simulink model "lump_cell_currentprofilev1_comparison"  (R2024b)
settings: Solver=FixedStepAuto  StartTime=0.0  StopTime=1320  FixedStep=0.001  RelTol=1e-3
model workspace (MAT data in the model file):
  A_busbar = 0.0015
  A_pack = 0.0059475
  C_nominal = 3
  I_max = 157.708978328
  P = 5
  S = 138
  SoC_initial = 0.769
  T_amb = 296.65
  W_max = 34
  busbar_CC_area = 0.000108
  busbar_Cp = 237
  busbar_length = 0.032
  busbar_mass = 0.01
  busbar_resistivity = 1.68e-08
  busbar_thermalcontact_resistance = 1
  cell_Cp = 1000
  cell_mass = 0.046
  h_busbar = 5
  h_pack = 5
settings Model: Creator=kara.28  LastModifiedBy=kara.28

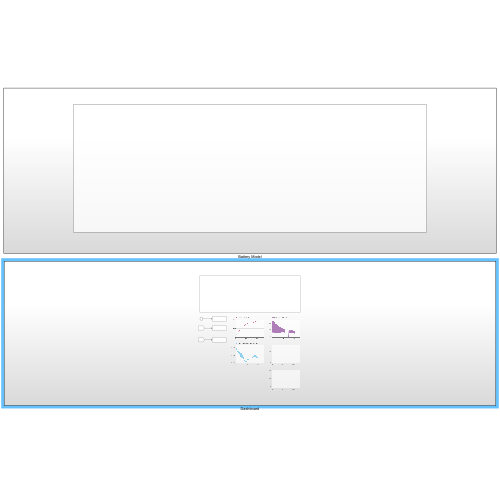
[thumbnail: Simulink's stored preview of the top-level diagram]
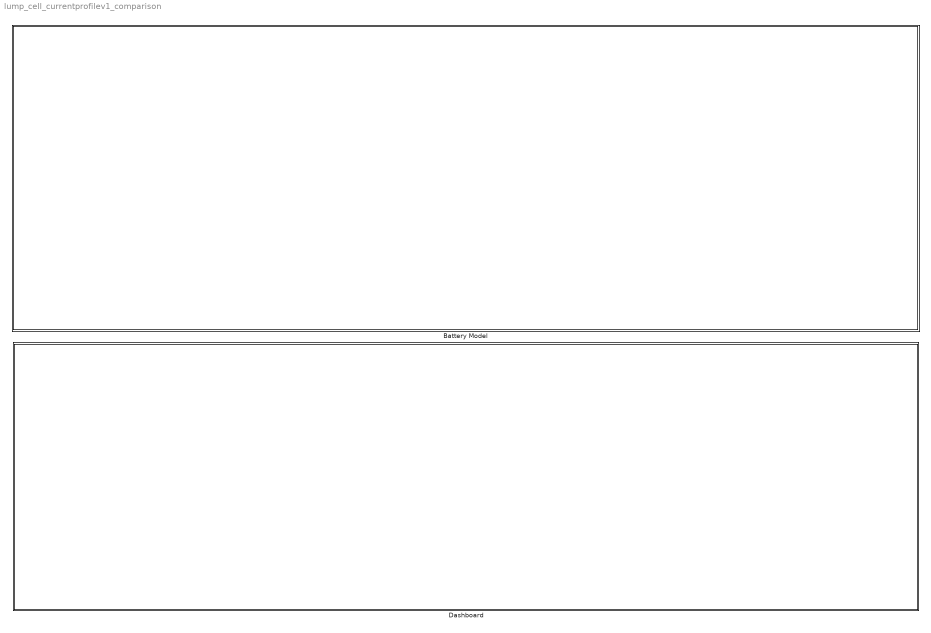
== system lump_cell_currentprofilev1_comparison ==
  Battery Model : Subsystem
  Dashboard : Subsystem

== system lump_cell_currentprofilev1_comparison/Battery Model ==
  Battery Cells : Subsystem

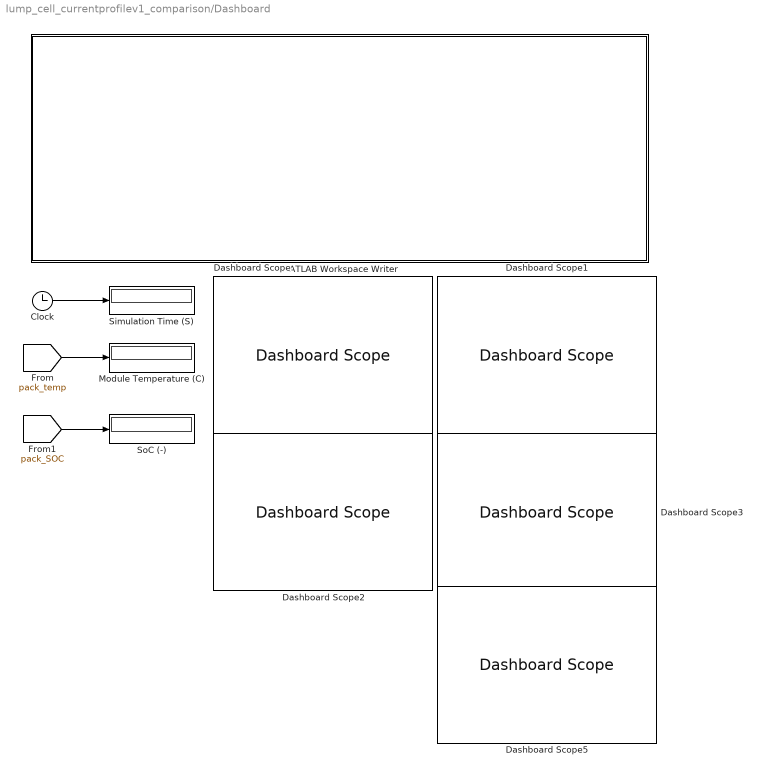
== system lump_cell_currentprofilev1_comparison/Dashboard ==
  Clock : Clock
  Dashboard Scope : DashboardScope  Ymin=35  Ymax=60
  Dashboard Scope1 : DashboardScope  Ymin=0  Ymax=180
  Dashboard Scope2 : DashboardScope
  Dashboard Scope3 : DashboardScope  Ymin=0  Ymax=1
  Dashboard Scope5 : DashboardScope
  MATLAB Workspace Writer : Subsystem
  Module Temperature (C) : Display
  Simulation Time (S) : Display
  SoC (-) : Display
  wires:
  Clock/1 -> Simulation Time (S)/1
  [pack_temp] -> Module Temperature (C)/1
  [pack_SOC] -> SoC (-)/1

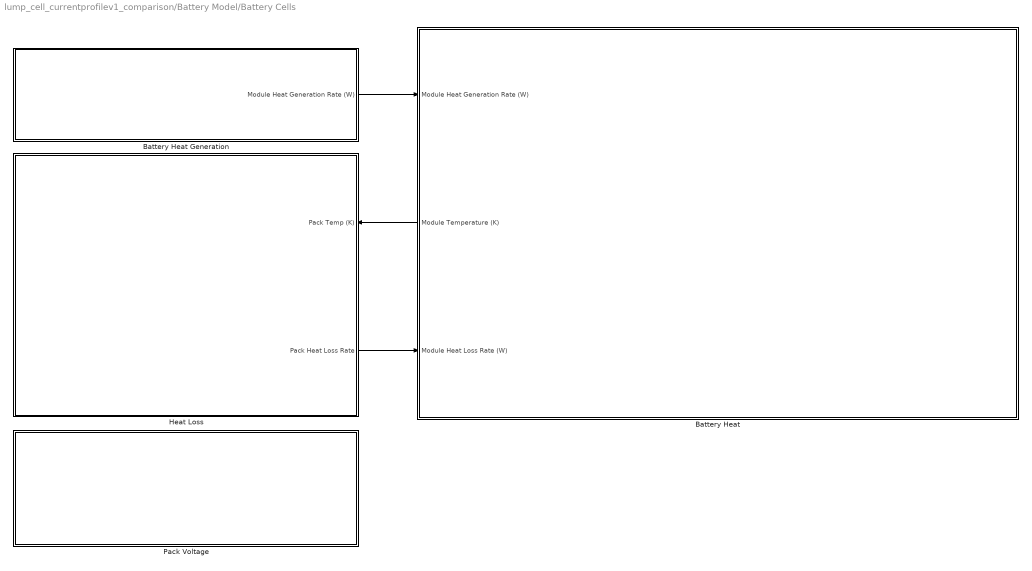
== system lump_cell_currentprofilev1_comparison/Battery Model/Battery Cells ==
  Battery Heat : Subsystem
      settings: PortSchema="{\"entries\":[{\"content\":{\"sides\":[{\"content\":{\"connectorIds\":[\"In1\",\"Out1\",\"In2\"]},\"type\":\"ConnectorPlacement.EquallySpacedRectSide\",\"uuid\":\"0f7c0562-63f7-413a-9c65-7d5d0f23ac53\"},{\"content\":{\"side\":\"RIGHT\"},\"type\":\"ConnectorPlacement.EquallySpacedRectSide\",\"uuid\":\"6856fc4a-e601-47fb-aafe-3183d6398fa2\"},{\"content\":{\"side\":\"TOP\"},\"type\":\"ConnectorPlacement.EquallySpacedRectSide\",\"uuid\":\"93500152-ab0c-4e86-a765-8796b82b9cd6\"}]},\"type\":\"ConnectorPlacement.EquallySpacedConnector\",\"uuid\":\"8bef09a8-0835-4033-ba4e-3f5f6277d0ac\"}],\"packageUris\":[\"http://schema.mathworks.com/mf0/Connector/R2020b\"],\"version\":\"1.0\"}"
  Battery Heat Generation : Subsystem
  Heat Loss : Subsystem
      settings: PortSchema="{\"entries\":[{\"content\":{\"sides\":[{\"content\":{},\"type\":\"ConnectorPlacement.EquallySpacedRectSide\",\"uuid\":\"cd11f8f0-ebc0-4dda-8c98-00f5919de41a\"},{\"content\":{\"connectorIds\":[\"In1\",\"Out1\"],\"side\":\"RIGHT\"},\"type\":\"ConnectorPlacement.EquallySpacedRectSide\",\"uuid\":\"2a68a9a1-bd97-4a17-8a8b-1aa98e9bd9a8\"},{\"content\":{\"side\":\"TOP\"},\"type\":\"ConnectorPlacement.EquallySpacedRectSide\",\"uuid\":\"debcc510-941b-4448-a371-f67c84c59f32\"}]},\"type\":\"ConnectorPlacement.EquallySpacedConnector\",\"uuid\":\"91559e46-754b-48b4-ac3e-ab135f9add0a\"}],\"packageUris\":[\"http://schema.mathworks.com/mf0/Connector/R2020b\"],\"version\":\"1.0\"}"
  Pack Voltage : Subsystem
  wires:
  Battery Heat/1(Module Temperature (K)) -> Heat Loss/1(Pack Temp (K))
  Battery Heat Generation/1(Module Heat Generation Rate (W)) -> Battery Heat/1(Module Heat Generation Rate (W))
  Heat Loss/1(Pack Heat Loss Rate) -> Battery Heat/2(Module Heat Loss Rate (W))

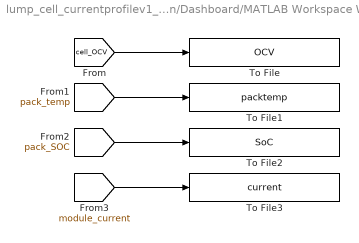
== system lump_cell_currentprofilev1_comparison/Dashboard/MATLAB Workspace Writer ==
  To File : ToFile  Filename=OCV  SampleTime=0.003
      settings: Decimation=3
  To File1 : ToFile  Filename=packtemp  SampleTime=0.003
      settings: Decimation=3
  To File2 : ToFile  Filename=SoC  SampleTime=0.003
      settings: Decimation=3
  To File3 : ToFile  Filename=current  SampleTime=0.003
      settings: Decimation=3
  wires:
  [module_current] -> To File3/1
  [cell_OCV] -> To File/1
  [pack_temp] -> To File1/1
  [pack_SOC] -> To File2/1

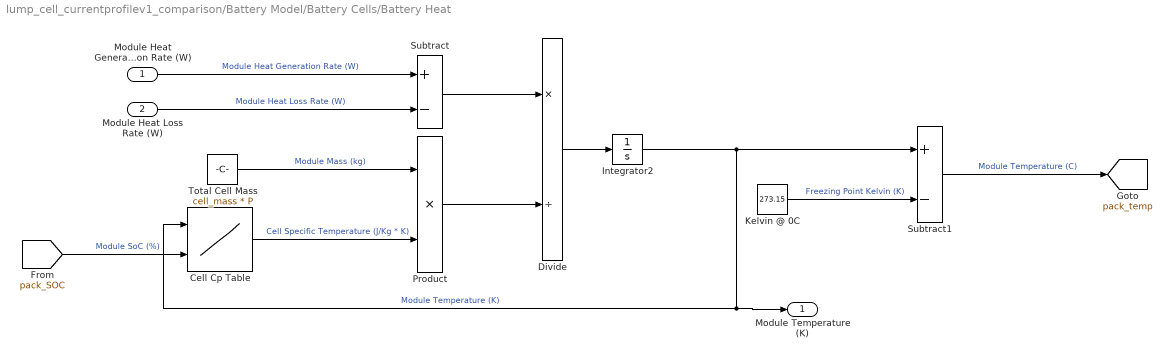
== system lump_cell_currentprofilev1_comparison/Battery Model/Battery Cells/Battery Heat ==
  Module Heat Generation Rate (W) : Inport
  Module Heat Loss Rate (W) : Inport  Port=2
  Cell Cp Table : Lookup_n-D  BreakpointsForDimension1=[296.0488;303.3425;312.147;321.5769;330.6423]  BreakpointsForDimension2=[0 0.5 1]  Table=[811.0868 819.6535 830.8545;814.1373 822.704 834.6964;817.9826 826.8129 838.6737000000001;822.2249 831.0552 843.4446;826.7299 835.8239 848.3459]  InterpMethod=Cubic spline  InternalRulePriority=Speed  RndMeth=Simplest
      settings: InputPortMap=u0,u1
  Divide : Product  Inputs=*/
  Integrator2 : Integrator  InitialCondition=T_amb
  Kelvin @ 0C : Constant  Value=273.15
  Product : Product
  Subtract : Sum  Inputs=+-
  Subtract1 : Sum  Inputs=+-
  Total Cell Mass : Constant  Value=cell_mass * P
  Module Temperature (K) : Outport
  tag scope: pack_temp=global
  wires:
  Cell Cp Table/1 -> Product/2  "Cell Specific Temperature (J/Kg * K)"
  Kelvin @ 0C/1 -> Subtract1/2  "Freezing Point Kelvin (K)"
  Divide/1 -> Integrator2/1
  Subtract/1 -> Divide/1
  Integrator2/1 -> Module Temperature (K)/1, Cell Cp Table/1, Subtract1/1  "Module Temperature (K)"
  Subtract1/1 -> [pack_temp]  "Module Temperature (C)"
  Total Cell Mass/1 -> Product/1  "Module Mass (kg)"
  Product/1 -> Divide/2
  Module Heat Loss Rate (W)/1 -> Subtract/2  "Module Heat Loss Rate (W)"
  Module Heat Generation Rate (W)/1 -> Subtract/1  "Module Heat Generation Rate (W)"
  [pack_SOC] -> Cell Cp Table/2  "Module SoC (%)"

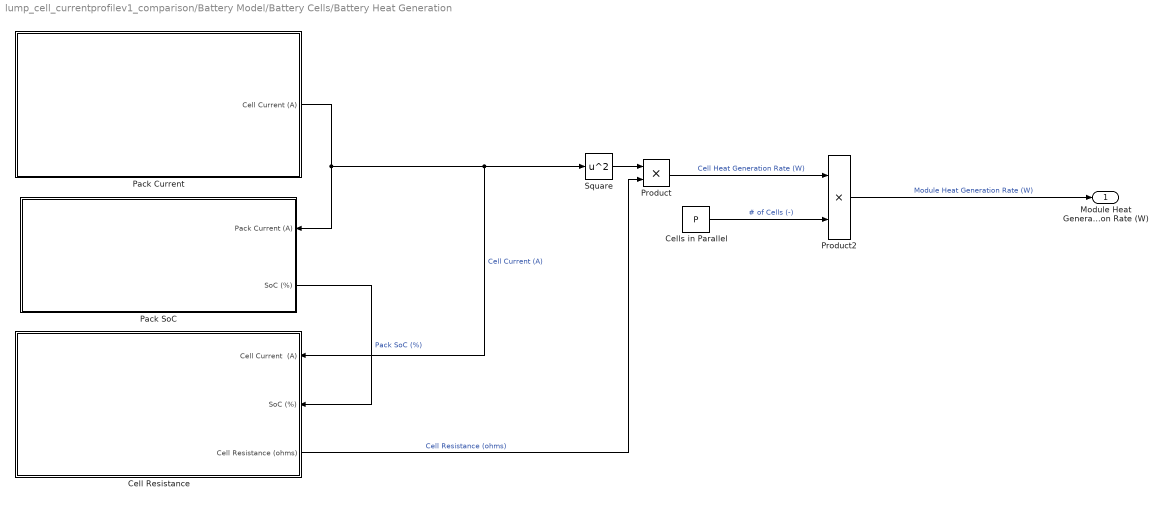
== system lump_cell_currentprofilev1_comparison/Battery Model/Battery Cells/Battery Heat Generation ==
  Cell Resistance : Subsystem
      settings: PortSchema="{\"entries\":[{\"content\":{\"sides\":[{\"content\":{},\"type\":\"ConnectorPlacement.EquallySpacedRectSide\",\"uuid\":\"1c6ff2a8-2c86-4b92-aa7d-5717a02d6f28\"},{\"content\":{\"connectorIds\":[\"In1\",\"In2\",\"Out1\"],\"side\":\"RIGHT\"},\"type\":\"ConnectorPlacement.EquallySpacedRectSide\",\"uuid\":\"52a4cb2c-e1db-459d-bd0a-206cc3bba6d1\"},{\"content\":{\"side\":\"TOP\"},\"type\":\"ConnectorPlacement.EquallySpacedRectSide\",\"uuid\":\"751bbbd6-abc7-4265-8d68-4aa70d69379f\"}]},\"type\":\"ConnectorPlacement.EquallySpacedConnector\",\"uuid\":\"b8f9630f-0167-4478-8d98-637e13782dcd\"}],\"packageUris\":[\"http://schema.mathworks.com/mf0/Connector/R2020b\"],\"version\":\"1.0\"}"
      mask Display: image('resistor.png');
  Cells in Parallel : Constant  Value=P
  Pack Current : Subsystem
      mask Display: image('current.png');
  Pack SoC : Subsystem
      settings: PortSchema="{\"entries\":[{\"content\":{\"sides\":[{\"content\":{},\"type\":\"ConnectorPlacement.EquallySpacedRectSide\",\"uuid\":\"1c6ff2a8-2c86-4b92-aa7d-5717a02d6f28\"},{\"content\":{\"connectorIds\":[\"In1\",\"Out1\"],\"side\":\"RIGHT\"},\"type\":\"ConnectorPlacement.EquallySpacedRectSide\",\"uuid\":\"52a4cb2c-e1db-459d-bd0a-206cc3bba6d1\"},{\"content\":{\"side\":\"TOP\"},\"type\":\"ConnectorPlacement.EquallySpacedRectSide\",\"uuid\":\"751bbbd6-abc7-4265-8d68-4aa70d69379f\"}]},\"type\":\"ConnectorPlacement.EquallySpacedConnector\",\"uuid\":\"b8f9630f-0167-4478-8d98-637e13782dcd\"}],\"packageUris\":[\"http://schema.mathworks.com/mf0/Connector/R2020b\"],\"version\":\"1.0\"}"
      mask Display: image('SoC.jpg');
  Product : Product
  Product2 : Product
  Square : Math  Operator=square
  Module Heat Generation Rate (W) : Outport
  wires:
  Pack Current/1(Cell Current (A)) -> Pack SoC/1(Pack Current (A)), Cell Resistance/1(Cell Current  (A)), Square/1  "Cell Current (A)"
  Cell Resistance/1(Cell Resistance (ohms)) -> Product/2  "Cell Resistance (ohms)"
  Square/1 -> Product/1
  Product/1 -> Product2/1  "Cell Heat Generation Rate (W)"
  Product2/1 -> Module Heat Generation Rate (W)/1  "Module Heat Generation Rate (W)"
  Pack SoC/1(SoC (%)) -> Cell Resistance/2(SoC (%))  "Pack SoC (%)"
  Cells in Parallel/1 -> Product2/2  "# of Cells (-)"

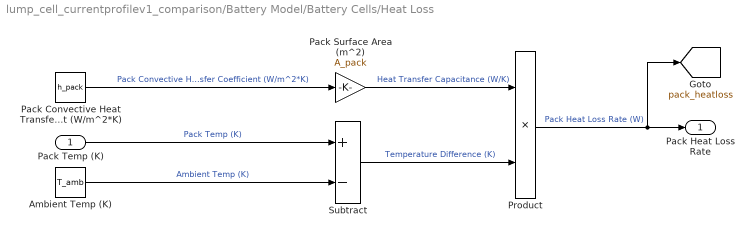
== system lump_cell_currentprofilev1_comparison/Battery Model/Battery Cells/Heat Loss ==
  Pack Temp (K) : Inport
  Ambient Temp (K) : Constant  Value=T_amb
  Pack Convective Heat Transfer Coefficient (W/m^2*K) : Constant  Value=h_pack
  Pack Surface Area (m^2) : Gain  Gain=A_pack
  Product : Product
  Subtract : Sum  Inputs=+-
  Pack Heat Loss Rate : Outport
  tag scope: pack_heatloss=global
  wires:
  Pack Convective Heat Transfer Coefficient (W/m^2*K)/1 -> Pack Surface Area (m^2)/1  "Pack Convective Heat Transfer Coefficient (W/m^2*K)"
  Subtract/1 -> Product/2  "Temperature Difference (K)"
  Pack Surface Area (m^2)/1 -> Product/1  "Heat Transfer Capacitance (W/K)"
  Product/1 -> [pack_heatloss], Pack Heat Loss Rate/1  "Pack Heat Loss Rate (W)"
  Pack Temp (K)/1 -> Subtract/1  "Pack Temp (K)"
  Ambient Temp (K)/1 -> Subtract/2  "Ambient Temp (K)"

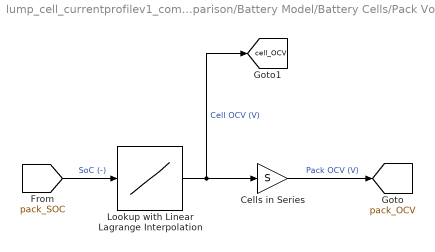
== system lump_cell_currentprofilev1_comparison/Battery Model/Battery Cells/Pack Voltage ==
  Cells in Series : Gain  Gain=S
  Lookup with Linear Lagrange Interpolation : Lookup_n-D  NumberOfTableDimensions=1  BreakpointsForDimension1=[0.100961;0.201247;0.30155;0.401865;0.502237;0.602602;0.7029339999999999;0.8032629999999999;0.903617;1]  Table=[3.227877;3.437376;3.537935;3.663634;3.755814;3.835423;3.940172;4.047017;4.097296;4.187904]  InterpMethod=Cubic spline  InternalRulePriority=Speed  RndMeth=Simplest
  tag scope: cell_OCV=global, pack_OCV=global
  wires:
  [pack_SOC] -> Lookup with Linear Lagrange Interpolation/1  "SoC (-)"
  Lookup with Linear Lagrange Interpolation/1 -> [cell_OCV], Cells in Series/1  "Cell OCV (V)"
  Cells in Series/1 -> [pack_OCV]  "Pack OCV (V)"

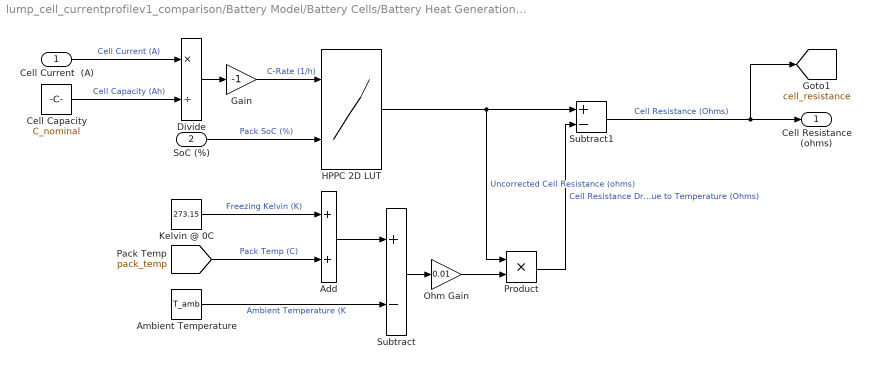
== system lump_cell_currentprofilev1_comparison/Battery Model/Battery Cells/Battery Heat Generation/Cell Resistance ==
  Cell Current  (A) : Inport
  SoC (%) : Inport  Port=2
  Add : Sum
  Ambient Temperature : Constant  Value=T_amb
  Cell Capacity : Constant  Value=C_nominal
  Divide : Product  Inputs=*/
  Gain : Gain  Gain=-1
  HPPC 2D LUT : Lookup_n-D  BreakpointsForDimension1=[-10;-5;-1;1;2;3]  BreakpointsForDimension2=[0.1;0.2;0.3;0.4;0.5;0.6;0.7;0.8;0.9;1]  Table=[0.018906 0.01868 0.018453 0.018226 0.017999 0.017916 0.017743 0.018183 0.019549 0.022703;0.021356 0.020344 0.019332 0.019017 0.018694 0.018598 0.018319 0.018773 0.020642 0.024917;0.02305 0.020909 0.018859 0.019644 0.019687 0.018989 0.018291 0.019295 0.021608 0.026536;0.023001 0.020599 0.019683 0.019161 0.01894 0.018506 0.018636 0.019336 0.020993 0.02265;0.022654 0.020712 0.018901 0.018682 0.018442 0.018289 0.017788 0.017286 0.016785 0.016283;0.019898 0.017891 0.017366 0.01725 0.01725 0.017251 0.017251 0.017251 0.017251 0.017251]  InterpMethod=Cubic spline  ExtrapMethod=Clip  InternalRulePriority=Speed  RndMeth=Simplest
      settings: InputPortMap=u0,u1
  Kelvin @ 0C : Constant  Value=273.15
  Ohm Gain : Gain  Gain=0.01
  Product : Product
  Subtract : Sum  Inputs=+-
  Subtract1 : Sum  Inputs=+-
  Cell Resistance (ohms) : Outport
  tag scope: cell_resistance=global
  wires:
  Cell Current  (A)/1 -> Divide/1  "Cell Current (A)"
  Cell Capacity/1 -> Divide/2  "Cell Capacity (Ah)"
  SoC (%)/1 -> HPPC 2D LUT/2  "Pack SoC (%)"
  HPPC 2D LUT/1 -> Subtract1/1, Product/1  "Uncorrected Cell Resistance (ohms)"
  Divide/1 -> Gain/1
  Gain/1 -> HPPC 2D LUT/1  "C-Rate (1/h)"
  Subtract/1 -> Ohm Gain/1
  Ambient Temperature/1 -> Subtract/2  "Ambient Temperature (K"
  [pack_temp] -> Add/2  "Pack Temp (C)"
  Add/1 -> Subtract/1
  Kelvin @ 0C/1 -> Add/1  "Freezing Kelvin (K)"
  Ohm Gain/1 -> Product/2
  Product/1 -> Subtract1/2  "Cell Resistance Drop Due to Temperature (Ohms)"
  Subtract1/1 -> [cell_resistance], Cell Resistance (ohms)/1  "Cell Resistance (Ohms)"

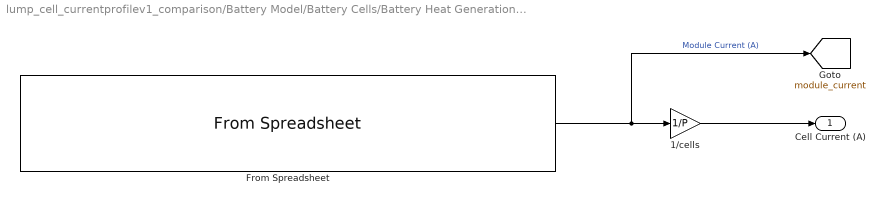
== system lump_cell_currentprofilev1_comparison/Battery Model/Battery Cells/Battery Heat Generation/Pack Current ==
  1/cells : Gain  Gain=1/P
  From Spreadsheet : FromSpreadsheet  FileName=C:\GITHUB\FB26_Controls\Battery Modeling\Simulink Model\Lump Model\V7\v1_current_profile_endurance.xlsx  SampleTime=-1
  Cell Current (A) : Outport
  tag scope: module_current=global
  wires:
  From Spreadsheet/1 -> [module_current], 1/cells/1  "Module Current (A)"
  1/cells/1 -> Cell Current (A)/1

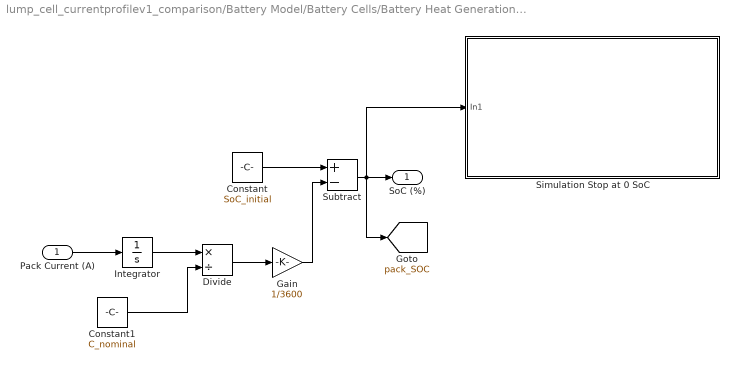
== system lump_cell_currentprofilev1_comparison/Battery Model/Battery Cells/Battery Heat Generation/Pack SoC ==
  Pack Current (A) : Inport
  Constant : Constant  Value=SoC_initial
  Constant1 : Constant  Value=C_nominal
  Divide : Product  Inputs=*/
  Gain : Gain  Gain=1/3600
  Integrator : Integrator
  Simulation Stop at 0 SoC : Subsystem
  Subtract : Sum  Inputs=+-
  SoC (%) : Outport
  tag scope: pack_SOC=global
  wires:
  Pack Current (A)/1 -> Integrator/1
  Constant/1 -> Subtract/1
  Integrator/1 -> Divide/1
  Subtract/1 -> Simulation Stop at 0 SoC/1(In1), [pack_SOC], SoC (%)/1
  Constant1/1 -> Divide/2
  Divide/1 -> Gain/1
  Gain/1 -> Subtract/2

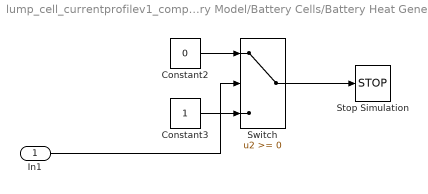
== system lump_cell_currentprofilev1_comparison/Battery Model/Battery Cells/Battery Heat Generation/Pack SoC/Simulation Stop at 0 SoC ==
  In1 : Inport
  Constant2 : Constant  Value=0
  Constant3 : Constant
  Stop Simulation : Stop
  Switch : Switch  SaturateOnIntegerOverflow=off  InputSameDT=off
  wires:
  Constant3/1 -> Switch/3
  Switch/1 -> Stop Simulation/1
  In1/1 -> Switch/2
  Constant2/1 -> Switch/1
